simulink model "dc_motor_control"  (R2017b)
settings: Solver=VariableStepAuto  StartTime=0.0  StopTime=5  RelTol=1e-3
values from neighbouring files (symbols this model uses):
  b = 0.1    [dc_motor_control_parameters.m]
  J = 0.01    [dc_motor_control_parameters.m]
  K = 0.01    [dc_motor_control_parameters.m]
  L = 0.5    [dc_motor_control_parameters.m]
  R = 1    [dc_motor_control_parameters.m]
settings Model: Creator=Damla  LastModifiedBy=dagac

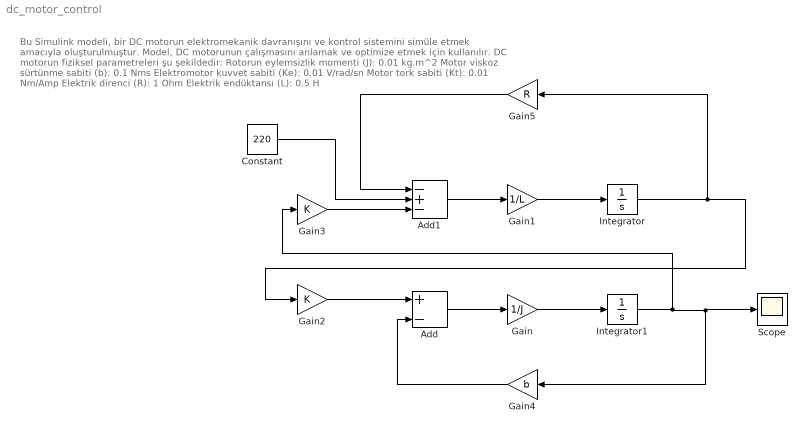
== system dc_motor_control ==
  note: Bu Simulink modeli, bir DC motorun elektromekanik davranışını ve kontrol sistemini simüle etmek amacıyla oluşturulmuştur.
      | Model, DC motorunun çalışmasını anlamak ve optimize etmek için kullanılır.
      |
      | DC motorun fiziksel parametreleri şu şekildedir:
      | Rotorun eylemsizlik momenti (J): 0.01 kg.m^2
      | Motor viskoz sürtünme sabiti (b): 0.1 Nms
      | Elektromotor kuvvet sabiti (Ke): 0.01 V/rad/sn
      | Motor tork sabiti (Kt): 0.01 Nm/Amp
      | Elektrik direnci (R): 1 Ohm
      | Elektrik endüktansı (L): 0.5 H
  Add : Sum  Inputs=+-
  Add1 : Sum  Inputs=-+-
  Constant : Constant  Value=220
  Gain : Gain  Gain=1/J
  Gain1 : Gain  Gain=1/L
  Gain2 : Gain  Gain=K
  Gain3 : Gain  Gain=K
  Gain4 : Gain  Gain=b
  Gain5 : Gain  Gain=R
  Integrator : Integrator
  Integrator1 : Integrator
  Scope : Scope
  wires:
  Gain1/1 -> Integrator/1
  Gain/1 -> Integrator1/1
  Add1/1 -> Gain1/1
  Add/1 -> Gain/1
  Gain3/1 -> Add1/3
  Gain2/1 -> Add/1
  Gain5/1 -> Add1/1
  Gain4/1 -> Add/2
  Integrator1/1 -> Gain4/1, Scope/1, Gain3/1
  Integrator/1 -> Gain2/1, Gain5/1
  Constant/1 -> Add1/2
